simulink model "project2_roomba_serialtest"  (R2017a)
settings: Solver=VariableStepAuto  StartTime=0.0  StopTime=Inf  RelTol=1e-3
libraries: martin_sean_RoombaLib x4, realtime_pacer_lib x1
settings Model: Creator=bai  LastModifiedBy=tuf53749

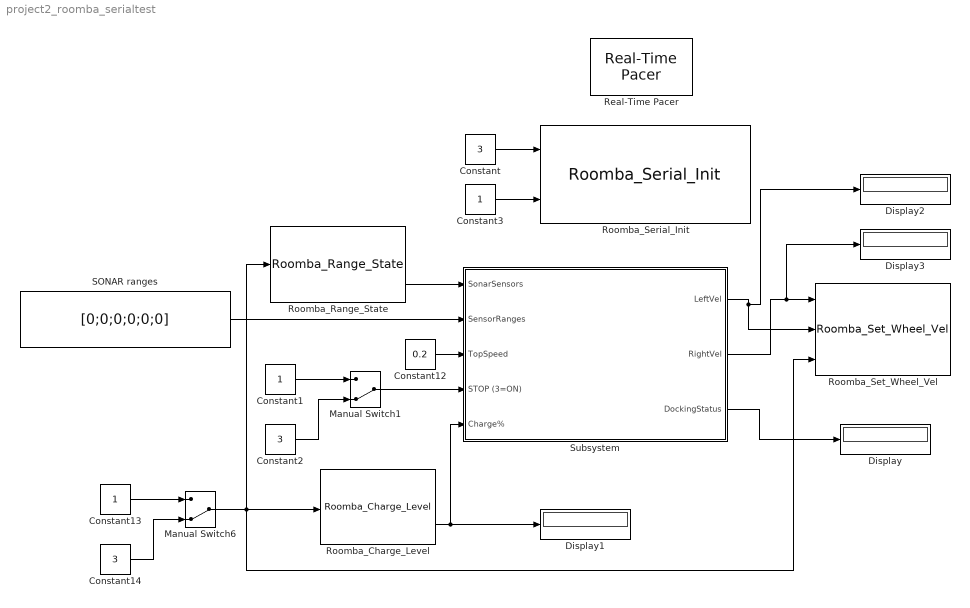
== system project2_roomba_serialtest ==
  Constant : Constant  Value=3
  Constant1 : Constant
  Constant12 : Constant  Value=0.2
  Constant13 : Constant
  Constant14 : Constant  Value=3
  Constant2 : Constant  Value=3
  Constant3 : Constant
  Display{,1..3} (4 alike) : Display
  Manual Switch1 : ManualSwitch  CurrentSetting=0
  Manual Switch6 : ManualSwitch  CurrentSetting=0
  Real-Time Pacer : realtime_pacer_lib/Real-Time Pacer  simTimePerRealTime=1
  Roomba_Charge_Level : martin_sean_RoombaLib/Roomba_Charge_Level  Description=Returns the battery charge level on the Roomba as a percentage. Updates every 100 seconds.
  Roomba_Range_State : martin_sean_RoombaLib/Roomba_Range_State  Description=|
      | Returns [1x6] array containing the state of the six IR sensors on the front of the Roomba. A 
      | '1' indicates there is an object ahead and a '0' indicates no object.
  Roomba_Serial_Init : martin_sean_RoombaLib/Roomba_Serial_Init  Description=|  Priority=-1000
      | Initializes a serial connection to the Roomba. Takes the COM Port number and mode as inputs.
      | For instance, COM Port = 3 and Mode = 1 will set up a connection to the Roomba on COM3
      | and place it in 'full' mode.
      | 
      | A 0 is returned after successful initialization.
  Roomba_Set_Wheel_Vel : martin_sean_RoombaLib/Roomba_Set_Wheel_Vel  Description=|
      | Sets the right and left wheel velocities on the Roomba. The values are in meters/sec between 
      | [-0.5, 0.5]. Negative velocity is backwards.
  SONAR ranges : Constant  Value=[0;0;0;0;0;0]
  Subsystem : Subsystem
  wires:
  Constant13/1 -> Manual Switch6/1
  Constant14/1 -> Manual Switch6/2
  Roomba_Range_State/2 -> Subsystem/1(SonarSensors)
  SONAR ranges/1 -> Subsystem/2(SensorRanges)
  Constant12/1 -> Subsystem/3(TopSpeed)
  Roomba_Charge_Level/2 -> Display1/1, Subsystem/5(Charge%)
  Manual Switch6/1 -> Roomba_Set_Wheel_Vel/3, Roomba_Range_State/1, Roomba_Charge_Level/1
  Constant1/1 -> Manual Switch1/1
  Constant2/1 -> Manual Switch1/2
  Manual Switch1/1 -> Subsystem/4(STOP (3=ON))
  Subsystem/2(RightVel) -> Display3/1, Roomba_Set_Wheel_Vel/1
  Subsystem/1(LeftVel) -> Display2/1, Roomba_Set_Wheel_Vel/2
  Subsystem/3(DockingStatus) -> Display/1
  Constant/1 -> Roomba_Serial_Init/1
  Constant3/1 -> Roomba_Serial_Init/2

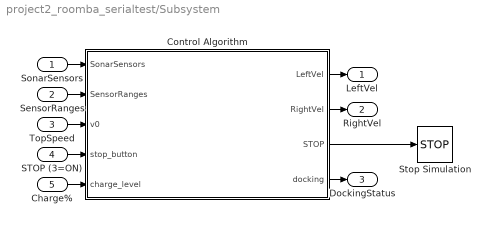
== system project2_roomba_serialtest/Subsystem ==
  SonarSensors : Inport
  SensorRanges : Inport  Port=2
  TopSpeed : Inport  Port=3
  STOP (3=ON) : Inport  Port=4
  Charge% : Inport  Port=5
  Control Algorithm : Stateflow chart  TreatAsAtomicUnit=on  mask{v0=1}
      mask prompts: v0 "Wheel Angular Velocity"
  Stop Simulation : Stop
  LeftVel : Outport
  RightVel : Outport  Port=2
  DockingStatus : Outport  Port=3
  wires:
  SonarSensors/1 -> Control Algorithm/1(SonarSensors)
  Charge%/1 -> Control Algorithm/5(charge_level)
  SensorRanges/1 -> Control Algorithm/2(SensorRanges)
  STOP (3=ON)/1 -> Control Algorithm/4(stop_button)
  Control Algorithm/1(LeftVel) -> LeftVel/1
  Control Algorithm/2(RightVel) -> RightVel/1
  TopSpeed/1 -> Control Algorithm/3(v0)
  Control Algorithm/4(docking) -> DockingStatus/1
  Control Algorithm/3(STOP) -> Stop Simulation/1

== stateflow chart project2_roomba_serialtest/Subsystem/Control Algorithm ==
  state BatteryLevelLogic [parallel]
    settings: executionOrder=3
    state CheckBat
      en:
      docking = 0;
    state LowBat
      en:
      docking = 1;
      SeekDockRoomba_Get();
    (default) -> CheckBat
    CheckBat -> LowBat : [charge_level <= 10]
  state EmergencyStopLogic [parallel]
    settings: executionOrder=1
    state StopButtonOFF
      en:
      %do nothing
      %
      STOP = 0;
    state StopButtonON
      en:
      LeftVel = 0;
      RightVel = 0;
      %this output must be
      %wired to Simulink
      %stop sink block
      %
      STOP = 1;
    (default) -> StopButtonOFF : {STOP=0;}
    StopButtonOFF -> StopButtonOFF [order 2] : after(0.1,sec)
    StopButtonOFF -> StopButtonON [order 1] : [stop_button == 3]
  state ObstacleAvoidLogic [parallel]
    en,du:
    frontSensors = SonarSensors(3:4);
    %frontSensors = SonarSensors(3:4) > SensorRanges(3:4);
    %leftMostSensors = [SonarSensors(1)] > SensorRanges(1);
    %leftMiddleSensors = [SonarSensors(1:2)] > SensorRanges(1:2);
    %rightMiddleSensors = [SonarSensors(5:6)] > SensorRanges(5:6);
    %rightMostSensors = [SonarSensors(6) ]> SensorRanges(6);
    leftMT=[SonarSensors(1)]; %>SensorRanges(1);
    leftMD=[SonarSensors(2)]; %>SensorRanges(2);
    leftFT=[SonarSensors(3)]; %>SensorRanges(3);
    rightFT=[SonarSensors(4)]; %>SensorRanges(4);
    rightMD=[SonarSensors(5)]; %>SensorRanges(5);
    rightMT=[SonarSensors(6)]; %>SensorRanges(6);
    settings: executionOrder=2
    state InitialCount
      en:
      count=0;
    state ReverseABit
      en,du:
      RightVel = -v0;
      LeftVel = -v0;
    state GoStraight
      en,du:
      RightVel = v0;
      LeftVel = v0;
    state TurnRightWide
      du:
      RightVel = v0/2;
      LeftVel = v0;
    state TurnRightTight
      du :
      RightVel = v0/5;
      LeftVel = v0;
    state TurnLeftInPlace
      du :
      RightVel = v0;
      LeftVel = -v0;
    state TurnRightInPlace
      du :
      RightVel = -v0;
      LeftVel = v0;
    state TurnLeftWide
      du :
      RightVel = v0;
      LeftVel = v0/2;
    state TurnLeftTight
      du :
      RightVel = v0;
      LeftVel = v0/5;
    state ReverseABit1
      en,du:
      RightVel = -v0;
      LeftVel = -v0;
    state ReverseALot
      en,du:
      RightVel = -v0;
      LeftVel = -v0;
    state DetermineRightLeft
    state DeterminerightWide
    state DetermineLeftTight
    state Nothing
    state DetermineCount
    state DeterminerightTight
    state DetermineFront
    state DetermineLeftWide
    state Count
      entry:count=count+1;
    state Stop
      en,du:
      RightVel = 0;
      LeftVel = 0;
    (default) -> InitialCount
    InitialCount -> ReverseABit
    ReverseABit -> GoStraight : after(3,sec)
    GoStraight -> DeterminerightWide
    TurnRightWide -> GoStraight : [leftMT<1]
    TurnRightTight -> GoStraight : [leftMT<1&&leftMD<1]
    TurnLeftInPlace -> GoStraight : [rightFT<1&&leftFT<1]
    TurnRightInPlace -> GoStraight : [rightFT<1&&leftFT<1]
    TurnLeftWide -> GoStraight : [rightMT<1]
    TurnLeftTight -> GoStraight : [rightMD<1&&rightMT<1]
    Nothing -> GoStraight [order 1] : [leftMT<1&&...
        | leftMD<1&&...
        | leftFT<1&&...
        | rightFT<1&&...
        | rightMD<1&&...
        | rightMT<1]
    ReverseABit1 -> GoStraight : after(2,sec)
    ReverseALot -> GoStraight : after(6,sec)
    DeterminerightTight -> TurnRightTight [order 1] : [leftMT>0&&...
        | leftMD>0&&...
        | leftFT<1&&...
        | rightFT<1&&...
        | rightMD<1&&...
        | rightMT<1]
    DetermineRightLeft -> TurnLeftInPlace [order 2] : %default
    DetermineRightLeft -> TurnRightInPlace [order 1] : [rightFT>rightMD]
    DetermineLeftWide -> TurnLeftWide [order 1] : [leftMT<1&&...
        | leftMD<1&&...
        | leftFT<1&&...
        | rightFT<1&&...
        | rightMD<1&&...
        | rightMT>0]
    DetermineLeftTight -> TurnLeftTight [order 1] : [leftMT<1&&...
        | leftMD<1&&...
        | leftFT<1&&...
        | rightFT<1&&...
        | rightMD>0&&...
        | rightMT>0]
    DeterminerightWide -> TurnRightWide [order 1] : [leftMT>0&&...
        | leftMD<1&&...
        | leftFT<1&&...
        | rightFT<1&&...
        | rightMD<1&&...
        | rightMT<1]
    DetermineCount -> ReverseABit1 [order 1] : [count<5]
    DetermineCount -> ReverseALot [order 3] : [count<10 && count>=5]
    DetermineFront -> DetermineRightLeft [order 1] : [leftMT<1&&...
        | leftMD<1&&leftFT>0&&...
        | rightFT>0&&rightMD<1&&...
        | rightMT<1]
    DeterminerightWide -> DeterminerightTight [order 2] : %default
    DetermineLeftTight -> Nothing [order 2] : %default
    DetermineLeftWide -> DetermineLeftTight [order 2] : %default
    Nothing -> Count [order 2] : %default
    Count -> DetermineCount : %default
    DetermineCount -> Stop [order 2] : [count>=10]
    DeterminerightTight -> DetermineFront [order 2] : %default
    DetermineFront -> DetermineLeftWide [order 2] : %default
  data: LeftVel output; RightVel output; SonarSensors input; frontSensors local; SensorRanges input; leftMostSensors local; leftMiddleSensors local; rightMostSensors local; rightMiddleSensors local; rightMT local; leftFT local; rightMD local; rightFT local; leftMD local; leftMT local; count local; v0 input [0..0.5]; stop_button input; STOP output [0..1]; charge_level input; docking output
  function SeekDockRoomba_Get:
    | function SeekDockRoomba_Get
    | persistent obj
    | coder.extrinsic('SeekDockRoomba');
    | coder.extrinsic('evalin');
    | coder.extrinsic('get');
    | if isempty(obj)
    |     obj = evalin('base','objWs');
    | end
    | SeekDockRoomba(obj);
